simulink model "exp2_2"  (R2013a)
settings: Solver=ode45  StartTime=0.0  StopTime=400  MaxStep=1  RelTol=1e-3
settings Model: Creator=kthammir  LastModifiedBy=wyh716
settings DataIOCC: SignalLoggingSaveFormat=ModelDataLogs
settings DebuggingCC: UnderspecifiedInitializationDetection=Simplified  MultiTaskDSMMsg=warning  MultiTaskCondExecSysMsg=none  StateNameClashWarn=none  StrictBusMsg=ErrorOnBusTreatedAsVector
settings RTWCC: IncludeERTFirstTime=on
settings GRTTargetCC: CodeReplacementLibrary=None  CPPClassGenCompliant=on

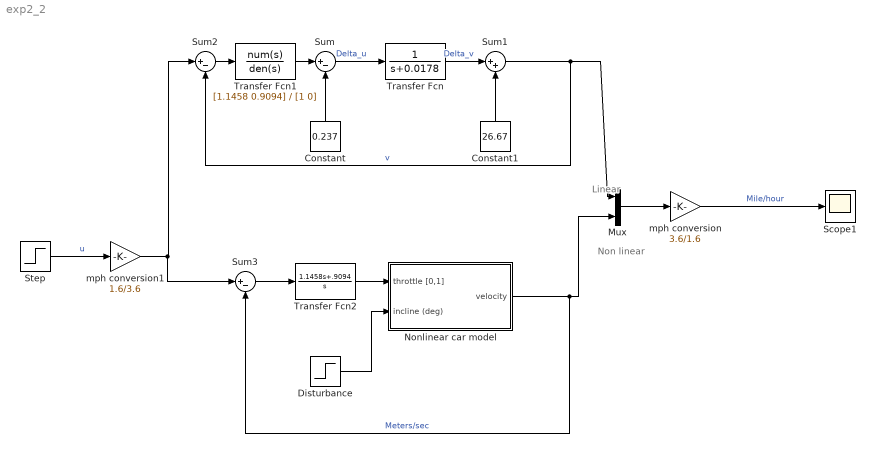
== system exp2_2 ==
  note: Non linear
  note: Linear
  Constant : Constant  Value=0.237
  Constant1 : Constant  Value=26.67
  Disturbance : Step  After=0  SampleTime=0
  Mux : Mux  Inputs=2
  Nonlinear car model : Subsystem  mask{ca=1*1500, cf=1*1500/55/55, m=1500}
      mask prompts: ca "acceleration coeff"; cf "friction/aero coeff"; m "mass"
  Scope1 : Scope
      settings: TimeRange=200  YMin=38.5  YMax=42.5
  Step : Step  Time=10  Before=60  After=65  SampleTime=0
  Sum : Sum  Inputs=|+-
  Sum1 : Sum  Inputs=|++
  Sum2 : Sum  Inputs=|+-
  Sum3 : Sum  Inputs=|+-
  Transfer Fcn : TransferFcn  Denominator=[1 0.0178]
  Transfer Fcn1 : TransferFcn  Numerator=[1.1458 0.9094]  Denominator=[1 0]
  Transfer Fcn2 : TransferFcn  Numerator=[1.1458 .9094]  Denominator=[1 0]
  mph conversion : Gain  Gain=3.6/1.6  SaturateOnIntegerOverflow=on  OutDataTypeStr=Inherit: Same as input  ParamDataTypeStr=Inherit: Same as input
  mph conversion1 : Gain  Gain=1.6/3.6  SaturateOnIntegerOverflow=on  OutDataTypeStr=Inherit: Same as input  ParamDataTypeStr=Inherit: Same as input
  wires:
  mph conversion/1 -> Scope1/1  "Mile/hour"
  Mux/1 -> mph conversion/1
  Nonlinear car model/1(velocity) -> Sum3/2, Mux/2  "Meters/sec"
  Sum/1 -> Transfer Fcn/1  "Delta_u"
  Transfer Fcn/1 -> Sum1/1  "Delta_v"
  Sum1/1 -> Sum2/2, Mux/1  "v"
  Constant/1 -> Sum/2
  Constant1/1 -> Sum1/2
  Step/1 -> mph conversion1/1  "u"
  Transfer Fcn1/1 -> Sum/1
  Sum2/1 -> Transfer Fcn1/1
  mph conversion1/1 -> Sum3/1, Sum2/1
  Transfer Fcn2/1 -> Nonlinear car model/1(throttle [0,1])
  Sum3/1 -> Transfer Fcn2/1
  Disturbance/1 -> Nonlinear car model/2(incline (deg))

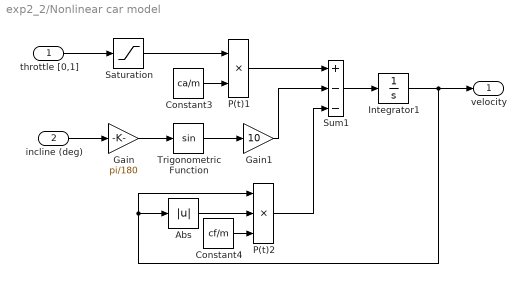
== system exp2_2/Nonlinear car model ==
  throttle [0,1] : Inport
  incline (deg) : Inport  Port=2
  Abs : Abs  SaturateOnIntegerOverflow=on
  Constant3 : Constant  Value=ca/m
  Constant4 : Constant  Value=cf/m
  Gain : Gain  Gain=pi/180  SaturateOnIntegerOverflow=on  OutDataTypeStr=Inherit: Same as input  ParamDataTypeStr=Inherit: Same as input
  Gain1 : Gain  Gain=10  SaturateOnIntegerOverflow=on  OutDataTypeStr=Inherit: Same as input  ParamDataTypeStr=Inherit: Same as input
  Integrator1 : Integrator  InitialCondition=26.67  UpperSaturationLimit=1  LowerSaturationLimit=0
  P(t)1 : Product  Inputs=**  SaturateOnIntegerOverflow=on  RndMeth=Zero  InputSameDT=on  OutDataTypeStr=Inherit: Same as first input
  P(t)2 : Product  Inputs=***  SaturateOnIntegerOverflow=on  RndMeth=Zero  InputSameDT=on  OutDataTypeStr=Inherit: Same as first input
  Saturation : Saturate  UpperLimit=3  LowerLimit=-1
  Sum1 : Sum  Inputs=+--  SaturateOnIntegerOverflow=on  InputSameDT=on  OutDataTypeStr=Inherit: Same as first input
  Trigonometric Function : Trigonometry
  velocity : Outport
  wires:
  Saturation/1 -> P(t)1/1
  Sum1/1 -> Integrator1/1
  Constant3/1 -> P(t)1/2
  P(t)1/1 -> Sum1/1
  Integrator1/1 -> Abs/1, P(t)2/1, velocity/1
  Constant4/1 -> P(t)2/3
  throttle [0,1]/1 -> Saturation/1
  incline (deg)/1 -> Gain/1
  P(t)2/1 -> Sum1/3
  Gain/1 -> Trigonometric Function/1
  Gain1/1 -> Sum1/2
  Trigonometric Function/1 -> Gain1/1
  Abs/1 -> P(t)2/2
